simulink model "simModell_jens"  (Simulink 9.0)
settings: Solver=ode45  StartTime=0.0  StopTime=simDauer  MaxStep=0.02  RelTol=1e-3  EnableMultiTasking=on
values from neighbouring files (symbols this model uses):
  beschlEnde = [4 0 0 4]    [Validierungsskript.m]
  beschlStaerke = [1.3 0 0 1.3]    [Validierungsskript.m]
  beschlStart = [2 0 0 2]    [Validierungsskript.m]
  bremsEnde = [10 0 0 17]    [Validierungsskript.m]
  bremsStaerke = [1.3 0 0 1.3]    [Validierungsskript.m]
  bremsStart = [8 0 0 15]    [Validierungsskript.m]
  rechteckSchwingAmplitude = [0 1.3 0 0]    [Validierungsskript.m]
  switchVar_recht_opt = [1 0 0 1]    [Validierungsskript.m]
settings Model: SuppressorTable=22 serialization::archive 11 0 6 0 0 0 11 0  Creator=beck  LastModifiedBy=jens
settings DataIOCC: LimitDataPoints=on  SignalLoggingSaveFormat=ModelDataLogs
settings OptimizationCC: ExpressionDepthLimit=2147483647  InitFltsAndDblsToZero=on
settings DebuggingCC: SaveWithParameterizedLinksMsg=none  SignalResolutionControl=TryResolveAllWithWarning  SolverPrmCheckMsg=warning  FcnCallInpInsideContextMsg=warning  StateNameClashWarn=warning  StrictBusMsg=Warning
settings GRTTargetCC: TargetFcnLib=ansi_tfl_tmw.mat  GeneratePreprocessorConditionals=Disable all  CombineOutputUpdateFcns=off  GRTInterface=on
settings ConfigComp: CovSFcnEnable=off

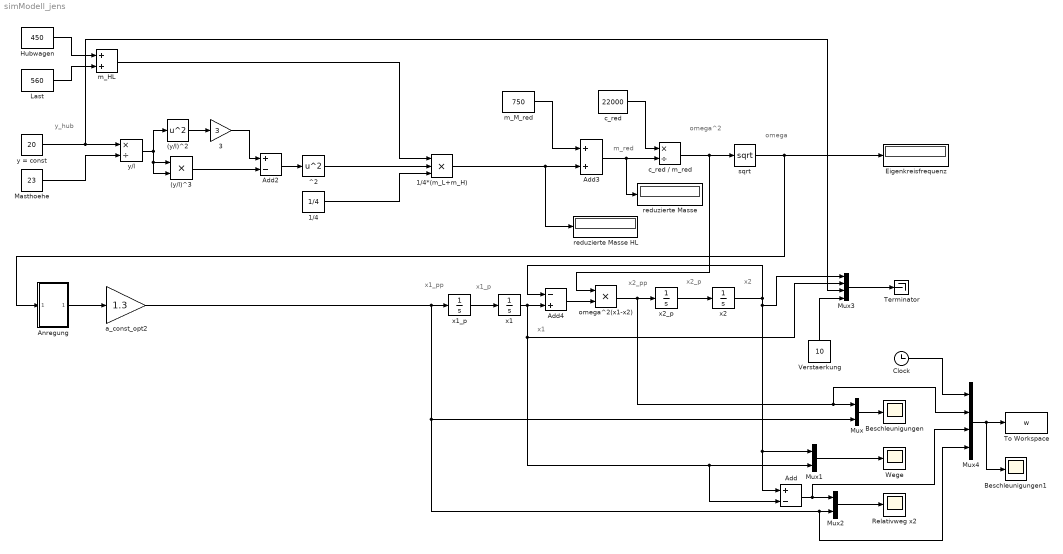
== system simModell_jens ==
  note: y_hub
  note: m_red
  note: omega^2
  note: x1_pp
  note: x2_pp
  note: x2_p
  note: x1_p
  note: omega
  note: x2
  note: x1
  (y/l)^2 : Math  Operator=square  SaturateOnIntegerOverflow=on
  (y/l)^3 : Product  RndMeth=Zero
  1/4 : Constant  Value=1/4
  1/4*(m_L+m_H) : Product  Inputs=3  RndMeth=Zero
  3 : Gain  Gain=3
  Add : Sum  Inputs=+-
  Add2 : Sum  Inputs=+-
  Add3 : Sum
  Add4 : Sum  Inputs=-+
  Anregung : Subsystem
  Beschleunigungen : Scope
  Beschleunigungen1 : Scope
  Clock : Clock
  Eigenkreisfrequenz : Display
  Hubwagen : Constant  Value=450
  Last : Constant  Value=560
  Masthoehe : Constant  Value=23
  Mux : Mux  Inputs=2
  Mux1 : Mux  Inputs=2
  Mux2 : Mux  Inputs=2
  Mux3 : Mux
  Mux4 : Mux
  Relativweg x2 : Scope
  Terminator : Terminator
  To Workspace : ToWorkspace  VariableName=w  SampleTime=-1
  Verstaerkung : Constant  Value=10
  Wege : Scope
  ^2 : Math  Operator=square  SaturateOnIntegerOverflow=on
  a_const_opt2 : Gain  Gain=1.3
  c_red : Constant  Value=22000
  c_red / m_red : Product  Inputs=*/  RndMeth=Zero
  m_HL : Sum
  m_M_red : Constant  Value=750
  omega^2(x1-x2) : Product  RndMeth=Zero
  reduzierte Masse : Display
      settings: Decimation=2
  reduzierte Masse HL : Display
      settings: Decimation=2
  sqrt : Math  Operator=sqrt  SaturateOnIntegerOverflow=on
  x1 : Integrator
  x1_p : Integrator
  x2 : Integrator
  x2_p : Integrator
  y = const : Constant  Value=20
  y/l : Product  Inputs=*/  RndMeth=Zero
  wires:
  y = const/1 -> y/l/1, Mux3/3
  Mux/1 -> Beschleunigungen/1
  Mux1/1 -> Wege/1
  Masthoehe/1 -> y/l/2
  (y/l)^2/1 -> 3/1
  3/1 -> Add2/1
  (y/l)^3/1 -> Add2/2
  y/l/1 -> (y/l)^3/2, (y/l)^3/1, (y/l)^2/1
  c_red/1 -> c_red / m_red/1
  c_red / m_red/1 -> sqrt/1, omega^2(x1-x2)/1
  Add3/1 -> reduzierte Masse/1, c_red / m_red/2
  sqrt/1 -> Eigenkreisfrequenz/1, Anregung/1(In1)
  omega^2(x1-x2)/1 -> x2_p/1, Mux/1, Mux4/2
  x2_p/1 -> x2/1
  x1_p/1 -> x1/1
  Add4/1 -> omega^2(x1-x2)/2
  x1/1 -> Add4/2, Mux1/2, Add/2, Mux3/2
  x2/1 -> Add4/1, Add/1, Mux1/1, Mux3/1
  Verstaerkung/1 -> Mux3/4
  Add2/1 -> ^2/1
  m_M_red/1 -> Add3/1
  Mux2/1 -> Relativweg x2/1
  Add/1 -> Mux2/1, Mux4/3
  Last/1 -> m_HL/2
  Hubwagen/1 -> m_HL/1
  1/4*(m_L+m_H)/1 -> Add3/2, reduzierte Masse HL/1
  ^2/1 -> 1/4*(m_L+m_H)/2
  m_HL/1 -> 1/4*(m_L+m_H)/1
  1/4/1 -> 1/4*(m_L+m_H)/3
  a_const_opt2/1 -> x1_p/1, Mux/2, Mux2/2, Mux4/4
  Anregung/1(Out1) -> a_const_opt2/1
  Clock/1 -> Mux4/1
  Mux4/1 -> To Workspace/1, Beschleunigungen1/1
  Mux3/1 -> Terminator/1

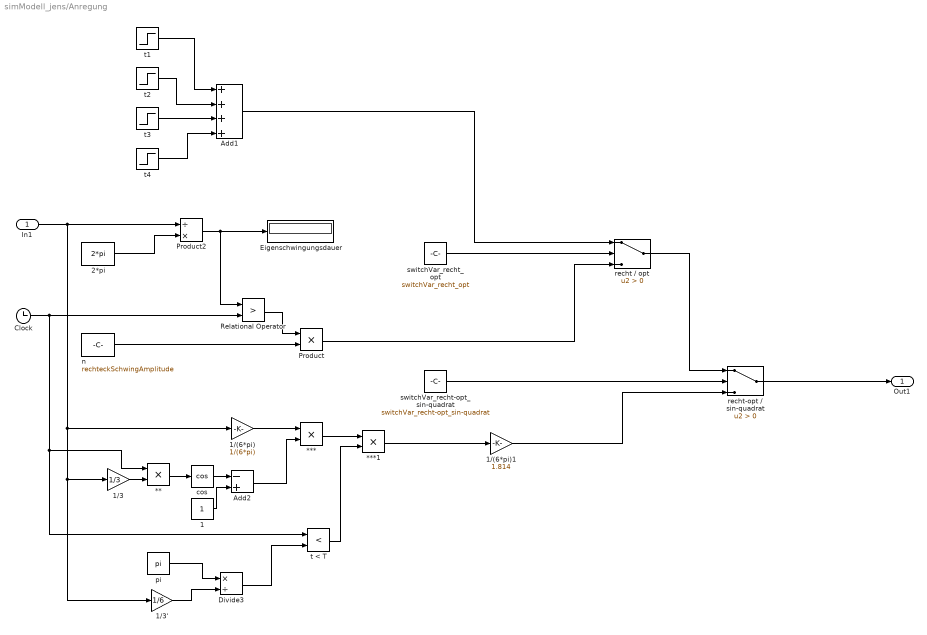
== system simModell_jens/Anregung ==
  In1 : Inport
  ** : Product  RndMeth=Zero
  *** : Product  RndMeth=Zero
  ***1 : Product  RndMeth=Zero
  1 : Constant
  1/(6*pi) : Gain  Gain=1/(6*pi)
  1/(6*pi)1 : Gain  Gain=1.814
  1/3 : Gain  Gain=1/3
  1/3' : Gain  Gain=1/6
  2*pi : Constant  Value=2*pi
  Add1 : Sum  Inputs=++++
  Add2 : Sum  Inputs=-+
  Clock : Clock
  Divide3 : Product  Inputs=*/
  Eigenschwingungsdauer : Display
  Product : Product  RndMeth=Zero
  Product2 : Product  Inputs=/*  RndMeth=Zero
  Relational Operator : RelationalOperator  Operator=>  RndMeth=Nearest
  "cos " : Trigonometry  Operator=cos
  n : Constant  Value=rechteckSchwingAmplitude
  pi : Constant  Value=pi
  recht / opt : Switch  Criteria=u2 > Threshold
  "recht-opt / sin-quadrat " : Switch  Criteria=u2 > Threshold
  switchVar_recht-opt_sin-quadrat : Constant  Value=switchVar_recht-opt_sin-quadrat
  switchVar_recht_opt : Constant  Value=switchVar_recht_opt
  t < T : RelationalOperator  Operator=<  OutDataTypeStr=boolean  RndMeth=Nearest
  t1 : Step  Time=beschlStart  SampleTime=0
  t2 : Step  Time=beschlEnde  After=-beschlStaerke  SampleTime=0
  t3 : Step  Time=bremsStart  After=bremsStaerke  SampleTime=0
  t4 : Step  Time=bremsEnde  After=-bremsStaerke  SampleTime=0
  Out1 : Outport
  wires:
  2*pi/1 -> Product2/2
  t1/1 -> Add1/1
  t2/1 -> Add1/2
  Clock/1 -> Relational Operator/2, **/1, t < T/1
  n/1 -> Product/2
  t3/1 -> Add1/3
  t4/1 -> Add1/4
  Product2/1 -> Eigenschwingungsdauer/1, Relational Operator/1
  Relational Operator/1 -> Product/1
  Product/1 -> recht / opt/3
  In1/1 -> Product2/1, 1/(6*pi)/1, 1/3/1, 1/3'/1
  1/3/1 -> **/2
  **/1 -> "cos "/1
  "cos "/1 -> Add2/1
  1/1 -> Add2/2
  1/(6*pi)/1 -> ***/1
  Add2/1 -> ***/2
  ***/1 -> ***1/1
  pi/1 -> Divide3/1
  Divide3/1 -> t < T/2
  t < T/1 -> ***1/2
  "recht-opt / sin-quadrat "/1 -> Out1/1
  1/3'/1 -> Divide3/2
  ***1/1 -> 1/(6*pi)1/1
  1/(6*pi)1/1 -> "recht-opt / sin-quadrat "/3
  Add1/1 -> recht / opt/1
  recht / opt/1 -> "recht-opt / sin-quadrat "/1
  switchVar_recht_opt/1 -> recht / opt/2
  switchVar_recht-opt_sin-quadrat/1 -> "recht-opt / sin-quadrat "/2
